simulink subsystem "DataLoader_Single_Array"  (R2019b)
settings: Solver=VariableStepAuto  StartTime=0.0  StopTime=10.0  RelTol=1e-3
settings Model: Creator=toons  LastModifiedBy=toons

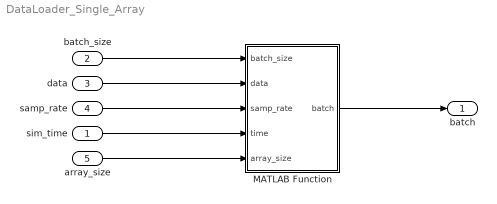
== system DataLoader_Single_Array ==
  sim_time : Inport
  batch_size : Inport  Port=2
  data : Inport  Port=3
  "samp_rate " : Inport  Port=4
  array_size : Inport  Port=5
  MATLAB Function : MATLAB Function  TreatAsAtomicUnit=on
  batch : Outport  SampleTime=0.02
  wires:
  batch_size/1 -> MATLAB Function/1(batch_size)
  data/1 -> MATLAB Function/2(data)
  "samp_rate "/1 -> MATLAB Function/3(samp_rate)
  sim_time/1 -> MATLAB Function/4(time)
  MATLAB Function/1(batch) -> batch/1
  array_size/1 -> MATLAB Function/5(array_size)

== matlab function DataLoader_Single_Array/MATLAB Function ==
  settings: updateMethod=DISCRETE  sampleTime=0.02
  data: batch_size input; batch output size=[batch_size array_size]; data input; samp_rate input; time input; array_size input
function batch = GetBatch(batch_size, data, samp_rate, time, array_size)
%GETBATCH Returns batch of samples of a lot more samples. 
%   INPUT:
%    - batch_size: number of samples you need to get of the data
%    - samp_rate_beam: sample rate 
%    - data: your big data chunk (which is not overcompensating anything)
%    _ time: current time in seconds
%   OUTPUT:
%    - batch: that sweet batch of data you requested. 
i_batch = max(ceil((samp_rate*time)/batch_size),1);
n_samples = size(data,1);

indx1 = (i_batch-1)*batch_size + 1;
indx2 = i_batch*batch_size;

batch = zeros(batch_size, array_size);
if indx1 > n_samples % return all zeros
    return
elseif indx2 > n_samples % zeropad the signal
    non_zero_data = data(indx1:n_samples,:);
    non_zero_size = size(non_zero_data,1);
    batch(1:non_zero_size,:) = non_zero_data;
    return
else
    batch = data(indx1:indx2,:);
    
end
